simulink model "initial_model1"  (R2017b)
settings: Solver=ode4  StartTime=0.0  StopTime=time_final  FixedStep=time_step  RelTol=1e-3  AbsTol=1e-6
values from neighbouring files (symbols this model uses):
  A_frontal = 2.8    [opt_output_torque_location1.mat]    (also in opt_output_torque_location1a.mat; tesla_sim_data1.m; tesla_sim_data1a.m)
  ap00 = -69.58    [opt_output_torque_location1.mat]    (also in opt_output_torque_location1a.mat; tesla_sim_data1.m; tesla_sim_data1a.m)
  ap01 = 11.22    [opt_output_torque_location1.mat]    (also in opt_output_torque_location1a.mat; tesla_sim_data1.m; tesla_sim_data1a.m)
  ap02 = -0.1665    [opt_output_torque_location1.mat]    (also in opt_output_torque_location1a.mat; tesla_sim_data1.m; tesla_sim_data1a.m)
  ap03 = 0.0006218    [opt_output_torque_location1.mat]    (also in opt_output_torque_location1a.mat; tesla_sim_data1.m; tesla_sim_data1a.m)
  ap10 = 0.5123    [opt_output_torque_location1.mat]    (also in opt_output_torque_location1a.mat; tesla_sim_data1.m; tesla_sim_data1a.m)
  ap11 = 0.009736    [opt_output_torque_location1.mat]    (also in opt_output_torque_location1a.mat; tesla_sim_data1.m; tesla_sim_data1a.m)
  ap12 = 0.0003316    [opt_output_torque_location1.mat]    (also in opt_output_torque_location1a.mat; tesla_sim_data1.m; tesla_sim_data1a.m)
  ap20 = -0.0007943    [opt_output_torque_location1.mat]    (also in opt_output_torque_location1a.mat; tesla_sim_data1.m; tesla_sim_data1a.m)
  ap21 = -4.587e-07    [opt_output_torque_location1.mat]    (also in opt_output_torque_location1a.mat; tesla_sim_data1.m; tesla_sim_data1a.m)
  ap30 = 3.794e-07    [opt_output_torque_location1.mat]    (also in opt_output_torque_location1a.mat; tesla_sim_data1.m; tesla_sim_data1a.m)
  C_d = 0.24    [opt_output_torque_location1.mat]    (also in opt_output_torque_location1a.mat; tesla_sim_data1.m; tesla_sim_data1a.m)
  enable_stop = 1    [opt_output_torque_location1.mat]    (also in opt_output_torque_location1a.mat; tesla_sim_data1.m; tesla_sim_data1a.m)
  ess_cap_scale = 1    [opt_output_torque_location1.mat]    (also in opt_output_torque_location1a.mat; tesla_sim_data1.m; tesla_sim_data1a.m)
  ess_fixtemp = 25    [opt_output_torque_location1.mat]    (also in opt_output_torque_location1a.mat; tesla_sim_data1.m; tesla_sim_data1a.m)
  ess_init_soc = soc_init_index(simrun)    [ev_sim_init1a.m]    (also in opt_output_torque_location1.mat = 0.6; opt_output_torque_location1a.mat = 0.6)
  ess_max_ah_cap = [257.142857143 257.142857143]    [opt_output_torque_location1.mat]    (also in opt_output_torque_location1a.mat; tesla_sim_data1.m = ess_max_kwhr_cap*1000/350*[1 1]; tesla_sim_data1a.m = ess_max_kwhr_cap*1000/350*[1 1])
  ess_max_volts = 9    [opt_output_torque_location1.mat]    (also in opt_output_torque_location1a.mat; tesla_sim_data1.m; tesla_sim_data1a.m)
  ess_min_volts = 6    [opt_output_torque_location1.mat]    (also in opt_output_torque_location1a.mat; tesla_sim_data1.m; tesla_sim_data1a.m)
  ess_module_num = 40    [opt_output_torque_location1.mat]    (also in opt_output_torque_location1a.mat; tesla_sim_data1.m; tesla_sim_data1a.m)
  ess_r_chg = [0.00235 0.00235 0.0022 0.0022 0.00205 0.00205 0.00198 0.00198 0.00198 0.00198 0.00196 0.00196 ... (22 elements, 2x11)]    [opt_output_torque_location1.mat]    (also in opt_output_torque_location1a.mat; tesla_sim_data1.m = [; tesla_sim_data1a.m = [)
  ess_r_dis = [0.00377 0.00377 0.00338 0.00338 0.003 0.003 0.0028 0.0028 0.00275 0.00275 0.00268 0.00268 ... (22 elements, 2x11)]    [opt_output_torque_location1.mat]    (also in opt_output_torque_location1a.mat; tesla_sim_data1.m = [; tesla_sim_data1a.m = [)
  ess_res_scale_coef = [1 0 1 0]    [opt_output_torque_location1.mat]    (also in opt_output_torque_location1a.mat; tesla_sim_data1.m; tesla_sim_data1a.m)
  ess_res_scale_fun =     [opt_output_torque_location1.mat]    (also in opt_output_torque_location1a.mat; tesla_sim_data1.m = inline('(x(1)*ess_module_num+x(2))/(x(3)*ess_cap_scale+x(4)); tesla_sim_data1a.m = inline('(x(1)*ess_module_num+x(2))/(x(3)*ess_cap_scale+x(4)))
  ess_soc = [0 0.1 0.2 0.3 0.4 0.5 0.6 0.7 0.8 0.9 1]    [opt_output_torque_location1.mat]    (also in opt_output_torque_location1a.mat; tesla_sim_data1.m; tesla_sim_data1a.m)
  ess_tmp = [0 25]    [opt_output_torque_location1.mat]    (also in opt_output_torque_location1a.mat; tesla_sim_data1.m; tesla_sim_data1a.m)
  ess_voc = [7.237 7.237 7.4047 7.4047 7.5106 7.5106 7.5873 7.5873 7.6459 7.6459 7.6909 7.6909 ... (22 elements, 2x11)]    [opt_output_torque_location1.mat]    (also in opt_output_torque_location1a.mat; tesla_sim_data1.m = [; tesla_sim_data1a.m = [)
  f_rolling = 0.018    [opt_output_torque_location1.mat]    (also in opt_output_torque_location1a.mat; tesla_sim_data1.m; tesla_sim_data1a.m)
  FR = 9.73    [opt_output_torque_location1.mat]    (also in opt_output_torque_location1a.mat; tesla_sim_data1.m; tesla_sim_data1a.m)
  g_gravity = 9.81    [opt_output_torque_location1.mat]    (also in opt_output_torque_location1a.mat; tesla_sim_data1.m; tesla_sim_data1a.m)
  K_lookup_real_pow = K_lookup_pow.*ones(d,d)    [tesla_sim_data1.m]
  Kp_c = 30    [ev_sim_init1a.m]    (also in opt_output_torque_location1.mat; opt_output_torque_location1a.mat)
  m_map_spd = [0 10.471975512 26.1799387799 52.3598775598 104.71975512 157.079632679 209.439510239 261.799387799 314.159265359 418.879020479 471.238898038 575.958653158 ... (17 elements, 1x17)]    [opt_output_torque_location1.mat]    (also in opt_output_torque_location1a.mat; tesla_sim_data1.m = [0	100	250	500	1000	1500	2000	2500	3000	4000	4500	5500	6000	; tesla_sim_data1a.m = [0	100	250	500	1000	1500	2000	2500	3000	4000	4500	5500	6000	)
  m_max_trq_IM = [329.46 329.46 329.46 329.46 329.46 329.46 329.46 329.46 329.46 329.46 329.46 329.46 ... (17 elements, 1x17)]    [opt_output_torque_location1.mat]    (also in opt_output_torque_location1a.mat; tesla_sim_data1.m = min(m_peak_trq_IM, m_peak_pwr*1000./m_map_spd); tesla_sim_data1a.m = min(m_peak_trq_IM, m_peak_pwr*1000./m_map_spd))
  m_max_trq_SR = [660.28 660.28 660.28 660.28 660.28 660.28 660.28 660.28 660.28 660.28 657.840431447 538.233080274 ... (17 elements, 1x17)]    [opt_output_torque_location1.mat]    (also in opt_output_torque_location1a.mat; tesla_sim_data1.m = min(m_peak_trq_SR, m_peak_pwr*1000./m_map_spd); tesla_sim_data1a.m = min(m_peak_trq_SR, m_peak_pwr*1000./m_map_spd))
  m_min_volts = 200    [opt_output_torque_location1.mat]    (also in opt_output_torque_location1a.mat; tesla_sim_data1.m; tesla_sim_data1a.m)
  m_peak_pwr = 310    [opt_output_torque_location1.mat]    (also in opt_output_torque_location1a.mat; tesla_sim_data1.m; tesla_sim_data1a.m)
  M_total = 2245.3052708    [opt_output_torque_location1.mat]    (also in opt_output_torque_location1a.mat; tesla_sim_data1.m; tesla_sim_data1a.m)
  mtr_speed_rad = [10 216.106176906 422.212353812 628.318530718]    [opt_output_torque_location1.mat]    (also in opt_output_torque_location1a.mat; tesla_sim_data1.m = linspace(0,6000*2*pi/60,d); tesla_sim_data1a.m = linspace(10,6000*2*pi/60,d))
  mtr_torque_Nm = [10 540 1070 1600]    [opt_output_torque_location1.mat]    (also in opt_output_torque_location1a.mat; tesla_sim_data1.m = linspace(0,1000,d); tesla_sim_data1a.m = linspace(10,1600,d))
  opt_output_power_location112 = [0 0.4 0.8 0.6 0.8 0 0.2 0.2 0.4 0.6 0 0.8 ... (25 elements, 5x5)]    [opt_output_power_location112.mat]
  p00 = -215.8    [opt_output_torque_location1.mat]    (also in opt_output_torque_location1a.mat; tesla_sim_data1.m; tesla_sim_data1a.m)
  p01 = 3.368    [opt_output_torque_location1.mat]    (also in opt_output_torque_location1a.mat; tesla_sim_data1.m; tesla_sim_data1a.m)
  p02 = -0.0178    [opt_output_torque_location1.mat]    (also in opt_output_torque_location1a.mat; tesla_sim_data1.m; tesla_sim_data1a.m)
  p03 = 6.515e-05    [opt_output_torque_location1.mat]    (also in opt_output_torque_location1a.mat; tesla_sim_data1.m; tesla_sim_data1a.m)
  p10 = 4.164    [opt_output_torque_location1.mat]    (also in opt_output_torque_location1a.mat; tesla_sim_data1.m; tesla_sim_data1a.m)
  p11 = 0.04408    [opt_output_torque_location1.mat]    (also in opt_output_torque_location1a.mat; tesla_sim_data1.m; tesla_sim_data1a.m)
  p12 = 9.874e-05    [opt_output_torque_location1.mat]    (also in opt_output_torque_location1a.mat; tesla_sim_data1.m; tesla_sim_data1a.m)
  p20 = -0.009417    [opt_output_torque_location1.mat]    (also in opt_output_torque_location1a.mat; tesla_sim_data1.m; tesla_sim_data1a.m)
  p21 = 5.981e-06    [opt_output_torque_location1.mat]    (also in opt_output_torque_location1a.mat; tesla_sim_data1.m; tesla_sim_data1a.m)
  p30 = 5.161e-06    [opt_output_torque_location1.mat]    (also in opt_output_torque_location1a.mat; tesla_sim_data1.m; tesla_sim_data1a.m)
  R_tire = 0.335    [opt_output_torque_location1.mat]    (also in opt_output_torque_location1a.mat; tesla_sim_data1.m; tesla_sim_data1a.m)
  regstop_soc = 0.9    [ev_sim_init1a.m]    (also in opt_output_torque_location1.mat; opt_output_torque_location1a.mat)
  rho_air = 1.2    [opt_output_torque_location1.mat]    (also in opt_output_torque_location1a.mat; tesla_sim_data1.m; tesla_sim_data1a.m)
  Ti_c = 60    [ev_sim_init1a.m]    (also in opt_output_torque_location1.mat; opt_output_torque_location1a.mat)
  time_final = 1*length(cyc_mph(:,2))    [ev_sim_init1a.m]
  Tt_c = 65    [ev_sim_init1a.m]    (also in opt_output_torque_location1.mat; opt_output_torque_location1a.mat)
  v_max_c = 100    [ev_sim_init1a.m]    (also in opt_output_torque_location1.mat; opt_output_torque_location1a.mat)
undefined symbols (not defined in the file or in its folder): cyc_mph
libraries: simulink x4
(part 2 of 2)

== system initial_model1/Rear IM/Torque Allocation Controller ==
  Input Speed : Inport
  Input Torque : Inport  Port=2
  Add2 : Sum
  Constant : Constant
  Efficiency TA Lookup : Lookup_n-D  BreakpointsForDimension1=mtr_torque_Nm  BreakpointsForDimension2=mtr_speed_rad  Table=K_lookup_real_pow  InterpMethod=Nearest  InternalRulePriority=Speed  RndMeth=Simplest  InputSameDT=on
  Scope : Scope
  K_out : Outport
  wires:
  Constant/1 -> Add2/1
  Efficiency TA Lookup/1 -> Add2/2
  Input Torque/1 -> Efficiency TA Lookup/1
  Input Speed/1 -> Efficiency TA Lookup/2
  Add2/1 -> Scope/1, K_out/1

== system initial_model1/Vehicle/Dynamics ==
  note: Assumptions:
      | 1. No loss
      | 2. Small pinion gear inertia
      | 3. Longitudinal dynamics only
  wheel speed (rad/s) : Inport
  Tm: motor torque (N/m) : Inport  Port=2
  "Tfb: friction brake torque (N/m) " : Inport  Port=3
  Aero Drag : Fcn  Expr=0.5*A_frontal*rho_air* C_d*u^2*R_tire^3/FR^2
  Constant : Constant
  Constant1 : Constant  Value=0
  Gain : Gain  Gain=FR  SaturateOnIntegerOverflow=on  OutDataTypeStr=Inherit: Same as input  ParamDataTypeStr=Inherit: Same as input
  Integrator1 : Integrator  InitialCondition=0.1  LimitOutput=on  LowerSaturationLimit=0.1
  Rolling Resistance : Fcn  Expr=M_total*g_gravity*f_rolling*R_tire*u
  Sum : Sum  Inputs=+---  SaturateOnIntegerOverflow=on
  Switch : Switch  Threshold=0.001  SaturateOnIntegerOverflow=on
  To Workspace3 : ToWorkspace  VariableName=T_fb  SampleTime=-1
  Vehicle Propulsion : Fcn  Expr=u/(M_total*R_tire^2/FR)
  motor speed (rad/s) : Outport  InitialOutput=0
  wires:
  Vehicle Propulsion/1 -> Integrator1/1
  Integrator1/1 -> motor speed (rad/s)/1, Aero Drag/1
  Rolling Resistance/1 -> Sum/3  "Roll Resis"
  Aero Drag/1 -> Sum/4
  wheel speed (rad/s)/1 -> Switch/2
  Tm: motor torque (N/m)/1 -> Gain/1  "Tm"
  Constant1/1 -> Switch/3
  Constant/1 -> Switch/1
  Switch/1 -> Rolling Resistance/1
  Gain/1 -> Sum/1
  "Tfb: friction brake torque (N/m) "/1 -> Sum/2, To Workspace3/1  "Tf"
  Sum/1 -> Vehicle Propulsion/1

== system initial_model1/Battery/pack Voc, Rint/Rchg (ohms) ==
  x0 : Inport
  y0 : Inport  Port=2
  Mux : Mux  Inputs=2
  S-function : S-Function  FunctionName=sftable2  Parameters=xindex, yindex, table  SFunctionDeploymentMode=off  EnableBusSupport=off
  table out : Outport  InitialOutput=0
  wires:
  y0/1 -> Mux/2
  S-function/1 -> table out/1
  x0/1 -> Mux/1
  Mux/1 -> S-function/1

== system initial_model1/Battery/pack Voc, Rint/Rdis (ohms) ==
  x0 : Inport
  y0 : Inport  Port=2
  Mux : Mux  Inputs=2
  S-function : S-Function  FunctionName=sftable2  Parameters=xindex, yindex, table  SFunctionDeploymentMode=off  EnableBusSupport=off
  table out : Outport  InitialOutput=0
  wires:
  y0/1 -> Mux/2
  S-function/1 -> table out/1
  x0/1 -> Mux/1
  Mux/1 -> S-function/1

== system initial_model1/Battery/pack Voc, Rint/VOC (V) ==
  x0 : Inport
  y0 : Inport  Port=2
  Mux : Mux  Inputs=2
  S-function : S-Function  FunctionName=sftable2  Parameters=xindex, yindex, table  SFunctionDeploymentMode=off  EnableBusSupport=off
  table out : Outport  InitialOutput=0
  wires:
  y0/1 -> Mux/2
  S-function/1 -> table out/1
  x0/1 -> Mux/1
  Mux/1 -> S-function/1

== system initial_model1/Hybrid Controller/Brake/Regen Control ==
  soc : Inport
  veh sped : Inport  Port=2
  Logical Operator : Logic  Inputs=3
  regen swith on : Constant
  soc < soc_stopcharging : Relay  OnSwitchValue=regstop_soc  OffSwitchValue=regstop_soc  OnOutputValue=0  OffOutputValue=1
  veh spd>= 0.4 mph : Relay  OnSwitchValue=0.4  OffSwitchValue=0.4
  "Use regen? " : Outport
  wires:
  veh sped/1 -> veh spd>= 0.4 mph/1
  soc/1 -> soc < soc_stopcharging/1
  veh spd>= 0.4 mph/1 -> Logical Operator/1
  Logical Operator/1 -> "Use regen? "/1
  soc < soc_stopcharging/1 -> Logical Operator/2
  regen swith on/1 -> Logical Operator/3
